simulink model "canon2"  (R2016a)
settings: Solver=VariableStepAuto  StartTime=0.0  StopTime=5.0  RelTol=1e-3
values from neighbouring files (symbols this model uses):
  A = 1    [canon2script.m]
  omega = 10    [canon2script.m]
  zeta = 0.1    [canon2script.m]
settings Model: Creator=kimtran  LastModifiedBy=kimtran
settings DataIOCC: SaveFormat=Array  Refine=4

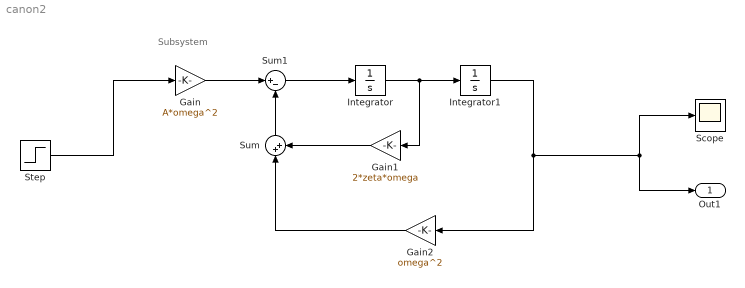
== system canon2 ==
  note: Subsystem
  Gain : Gain  Gain=A*omega^2
  Gain1 : Gain  Gain=2*zeta*omega
  Gain2 : Gain  Gain=omega^2
  Integrator : Integrator
  Integrator1 : Integrator
  Scope : Scope
  Step : Step  Time=0  SampleTime=0
  Sum : Sum  Inputs=|++
  Sum1 : Sum  Inputs=|+-
  Out1 : Outport
  wires:
  Integrator1/1 -> Out1/1, Scope/1, Gain2/1
  Gain/1 -> Sum1/1
  Gain1/1 -> Sum/2
  Step/1 -> Gain/1
  Integrator/1 -> Gain1/1, Integrator1/1
  Sum/1 -> Sum1/2
  Sum1/1 -> Integrator/1
  Gain2/1 -> Sum/1
